simulink model "test_sim"  (Simulink 10.3)
settings: Solver=FixedStepAuto  StartTime=0.0  StopTime=3  FixedStep=0.0001  RelTol=1e-3  EnableMultiTasking=on
settings Model: Creator=ljk  LastModifiedBy=fu  ExtModeTrigMode=oneshot  ExtModeArmWhenConnect=off
settings OptimizationCC: BlockReduction=off  BooleanDataType=off
settings DebuggingCC: SaveWithParameterizedLinksMsg=none  SignalResolutionControl=TryResolveAllWithWarning  MultiTaskDSMMsg=warning  MultiTaskCondExecSysMsg=none
settings HardwareCC: TargetUnknown=on

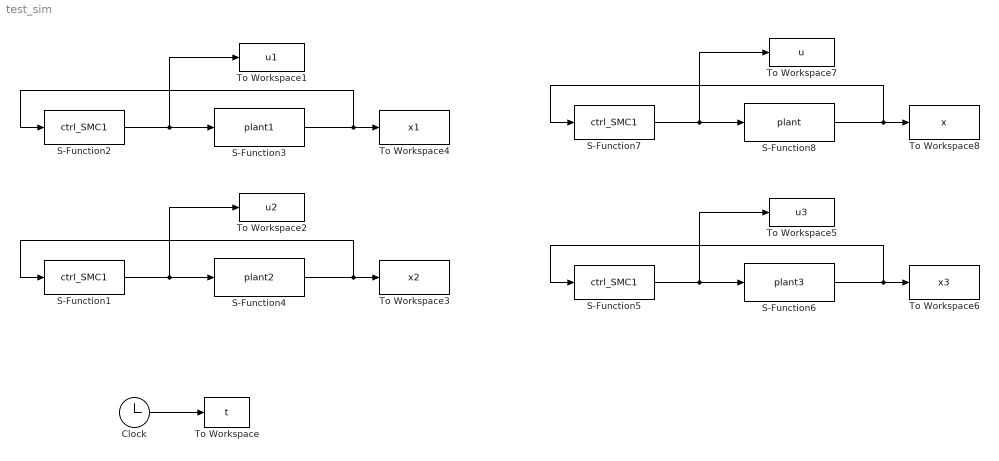
== system test_sim ==
  Clock : Clock
  S-Function{1..2,5,7} (4 alike) : S-Function  FunctionName=ctrl_SMC1  SFunctionDeploymentMode=off  EnableBusSupport=off
  S-Function3 : S-Function  FunctionName=plant1  SFunctionDeploymentMode=off  EnableBusSupport=off
  S-Function4 : S-Function  FunctionName=plant2  SFunctionDeploymentMode=off  EnableBusSupport=off
  S-Function6 : S-Function  FunctionName=plant3  SFunctionDeploymentMode=off  EnableBusSupport=off
  S-Function8 : S-Function  FunctionName=plant  SFunctionDeploymentMode=off  EnableBusSupport=off
  To Workspace : ToWorkspace  VariableName=t  SampleTime=-1
  To Workspace1 : ToWorkspace  VariableName=u1  SampleTime=-1
  To Workspace2 : ToWorkspace  VariableName=u2  SampleTime=-1
  To Workspace3 : ToWorkspace  VariableName=x2  SampleTime=-1
  To Workspace4 : ToWorkspace  VariableName=x1  SampleTime=-1
  To Workspace5 : ToWorkspace  VariableName=u3  SampleTime=-1
  To Workspace6 : ToWorkspace  VariableName=x3  SampleTime=-1
  To Workspace7 : ToWorkspace  VariableName=u  SampleTime=-1
  To Workspace8 : ToWorkspace  VariableName=x  SampleTime=-1
  wires:
  Clock/1 -> To Workspace/1
  S-Function3/1 -> S-Function2/1, To Workspace4/1
  S-Function2/1 -> S-Function3/1, To Workspace1/1
  S-Function1/1 -> S-Function4/1, To Workspace2/1
  S-Function4/1 -> S-Function1/1, To Workspace3/1
  S-Function5/1 -> S-Function6/1, To Workspace5/1
  S-Function6/1 -> S-Function5/1, To Workspace6/1
  S-Function8/1 -> S-Function7/1, To Workspace8/1
  S-Function7/1 -> S-Function8/1, To Workspace7/1
